simulink model "Progetto_Nostro_Defi"  (Simulink 8.6)
settings: Solver=ode45  StartTime=0.0  StopTime=2.7  RelTol=1e-3
values from neighbouring files (symbols this model uses):
  b = 1e-3    (= 0.001)    [motore_as_param.m]
  Edc = 700    [motore_as_param.m]
  J = Jc+Jm    (= 0.0532)    [motore_as_param.m]
  Kc = Cn/Wn-b    (= 0.178049310978)    [motore_as_param.m]
  Ki_i = 7664    [motore_as_param.m]
  Kp_i = Ki_i*tau_i    (= 32.018926058)    [motore_as_param.m]
  Lr = 123.95e-3    (= 0.12395)    [motore_as_param.m]
  Lrn = Lr    (= 0.12395)    [motore_as_param.m]
  Ls = 123.95e-3    (= 0.12395)    [motore_as_param.m]
  Lsn = Ls    (= 0.12395)    [motore_as_param.m]
  M = 118e-3    (= 0.118)    [motore_as_param.m]
  Mn = M    (= 0.118)    [motore_as_param.m]
  Nn = 1440    [motore_as_param.m]
  p = 2    [motore_as_param.m]
  Rr = 1.137    [motore_as_param.m]
  Rrn = Rr    (= 1.137)    [motore_as_param.m]
  Rs = 2.78    [motore_as_param.m]
  sigma = 1-M*M/(Ls*Lr)    (= 0.0937021444027)    [motore_as_param.m]
  sigman = 1-Mn*Mn/(Lsn*Lrn)    (= 0.0937021444027)    [motore_as_param.m]
  Tc = 200e-6    (= 0.0002)    [motore_as_param.m]
undefined symbols (not defined in the file): Imax, Ki_w, tau_w
libraries: simulink_need_slupdate x2, simulink x1
settings Model: Creator=Gian Filippo Rosi  LastModifiedBy=Gian Filippo Rosi
settings DataIOCC: LimitDataPoints=off  SaveOutput=off  SignalLogging=off  SaveTime=off
settings OptimizationCC: BooleanDataType=off  ExpressionDepthLimit=128  InitFltsAndDblsToZero=on
settings DebuggingCC: SaveWithParameterizedLinksMsg=none  SignalResolutionControl=TryResolveAllWithWarning  SolverPrmCheckMsg=none  MultiTaskDSMMsg=warning  MultiTaskCondExecSysMsg=none  FcnCallInpInsideContextMsg=UseLocalSettings  StateNameClashWarn=none
settings HardwareCC: TargetUnknown=on
settings GRTTargetCC: TargetFcnLib=ansi_tfl_tmw.mat  GeneratePreprocessorConditionals=Use local settings

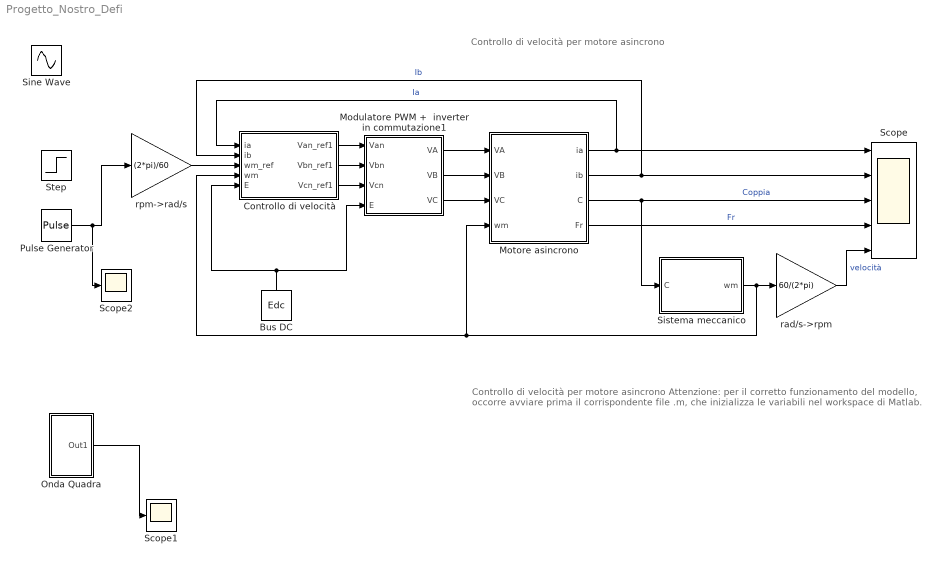
== system Progetto_Nostro_Defi ==
  note: Controllo di velocità per motore asincrono
  note: Controllo di velocità per motore asincrono
      |
      | Attenzione: per il corretto funzionamento del modello, occorre avviare prima
      | il corrispondente file .m, che inizializza le variabili nel workspace di Matlab.
  Bus DC : Constant  Value=Edc
  Controllo di velocità : Subsystem
  Modulatore PWM +  inverter in commutazione1 : Subsystem
  Motore asincrono : Subsystem
  Onda Quadra : Subsystem
  Pulse Generator : DiscretePulseGenerator  PulseType=Time based  Amplitude=2*Nn  PulseWidth=50  PhaseDelay=0.7
  Scope : Scope  NumInputPorts=5
  Scope1 : Scope
  Scope2 : Scope
  Sine Wave : Sin  Amplitude=Nn/4  Frequency=6.28  SampleTime=0
  Sistema meccanico : Subsystem
  Step : Step  Time=0.1+0.6  After=Nn  SampleTime=0
  rad/s->rpm : Gain  Gain=60/(2*pi)  SaturateOnIntegerOverflow=on  OutDataTypeStr=Inherit: Same as input  ParamDataTypeStr=Inherit: Same as input
  rpm->rad/s : Gain  Gain=(2*pi)/60  SaturateOnIntegerOverflow=on  OutDataTypeStr=Inherit: Same as input  ParamDataTypeStr=Inherit: Same as input
  wires:
  Motore asincrono/3(C) -> Scope/3, Sistema meccanico/1(C)  "Coppia"
  Sistema meccanico/1(wm) -> rad/s->rpm/1, Motore asincrono/4(wm), Controllo di velocità/4(wm)
  Motore asincrono/1(ia) -> Controllo di velocità/1(ia), Scope/1  "Ia"
  Motore asincrono/2(ib) -> Scope/2, Controllo di velocità/2(ib)  "Ib"
  Modulatore PWM +  inverter in commutazione1/1(VA) -> Motore asincrono/1(VA)
  Modulatore PWM +  inverter in commutazione1/2(VB) -> Motore asincrono/2(VB)
  Modulatore PWM +  inverter in commutazione1/3(VC) -> Motore asincrono/3(VC)
  Bus DC/1 -> Controllo di velocità/5(E), Modulatore PWM +  inverter in commutazione1/4(E)
  Controllo di velocità/1(Van_ref1) -> Modulatore PWM +  inverter in commutazione1/1(Van)
  Controllo di velocità/2(Vbn_ref1) -> Modulatore PWM +  inverter in commutazione1/2(Vbn)
  rpm->rad/s/1 -> Controllo di velocità/3(wm_ref)
  Controllo di velocità/3(Vcn_ref1) -> Modulatore PWM +  inverter in commutazione1/3(Vcn)
  rad/s->rpm/1 -> Scope/5  "velocità"
  Motore asincrono/4(Fr) -> Scope/4  "Fr"
  Onda Quadra/1(Out1) -> Scope1/1
  Pulse Generator/1 -> Scope2/1, rpm->rad/s/1

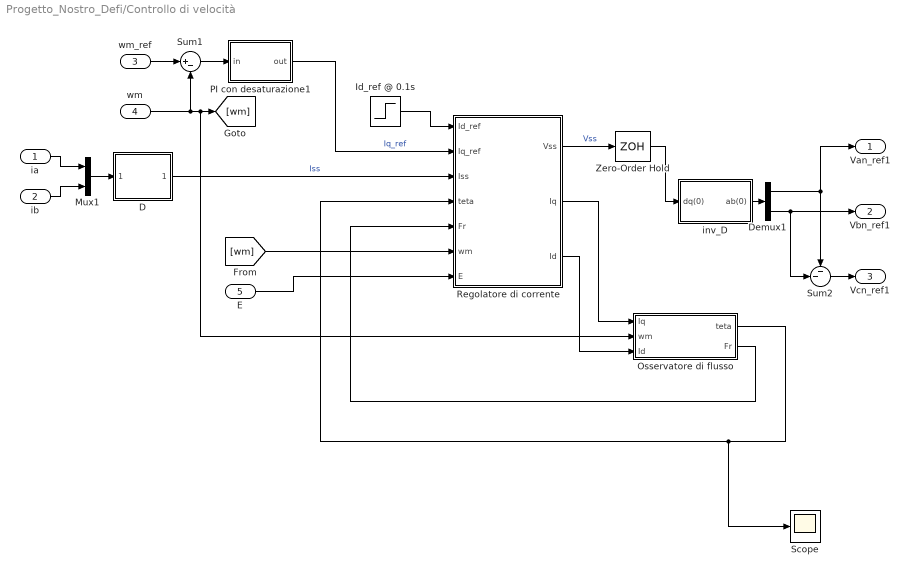
== system Progetto_Nostro_Defi/Controllo di velocità ==
  ia : Inport
  ib : Inport  Port=2
  wm_ref : Inport  Port=3
  wm : Inport  Port=4
  E : Inport  Port=5
  D : Subsystem
  Demux1 : Demux  Outputs=2
  Id_ref @ 0.1s : Step  Time=0.1  After=7.644  SampleTime=0
  Mux1 : Mux  Inputs=2
  Osservatore di flusso : Subsystem
  PI con desaturazione1 : Subsystem  mask{UB=Imax, LB=-Imax, tau=tau_w, Kp=Ki_w*tau_w}
      mask prompts: UB "Limite superiore"; LB "Limte inferiore"; tau "Tau (s)"
      mask Display: fprintf('PI\nantiwindup')
  Regolatore di corrente : Subsystem
  Scope : Scope
  Sum1 : Sum  Inputs=|+-
  Sum2 : Sum  Inputs=--|
  Zero-Order Hold : ZeroOrderHold  SampleTime=Tc
  inv_D : Subsystem
  Van_ref1 : Outport
  Vbn_ref1 : Outport  Port=2
  Vcn_ref1 : Outport  Port=3
  wires:
  inv_D/1(ab(0)) -> Demux1/1
  Sum2/1 -> Vcn_ref1/1
  Demux1/1 -> Sum2/1, Van_ref1/1
  Demux1/2 -> Sum2/2, Vbn_ref1/1
  Mux1/1 -> D/1(ab(c))
  ia/1 -> Mux1/1
  ib/1 -> Mux1/2
  D/1(dq(0)) -> Regolatore di corrente/3(Iss)  "Iss"
  Regolatore di corrente/1(Vss) -> Zero-Order Hold/1  "Vss"
  Osservatore di flusso/2(Fr) -> Regolatore di corrente/5(Fr)
  Osservatore di flusso/1(teta) -> Scope/1, Regolatore di corrente/4(teta)
  [wm] -> Regolatore di corrente/6(wm)
  E/1 -> Regolatore di corrente/7(E)
  wm/1 -> Osservatore di flusso/2(wm), [wm], Sum1/2
  wm_ref/1 -> Sum1/1
  Sum1/1 -> PI con desaturazione1/1(in)
  PI con desaturazione1/1(out) -> Regolatore di corrente/2(Iq_ref)  "Iq_ref"
  Zero-Order Hold/1 -> inv_D/1(dq(0))
  Id_ref @ 0.1s/1 -> Regolatore di corrente/1(Id_ref)
  Regolatore di corrente/2(Iq) -> Osservatore di flusso/1(Iq)
  Regolatore di corrente/3(Id) -> Osservatore di flusso/3(Id)

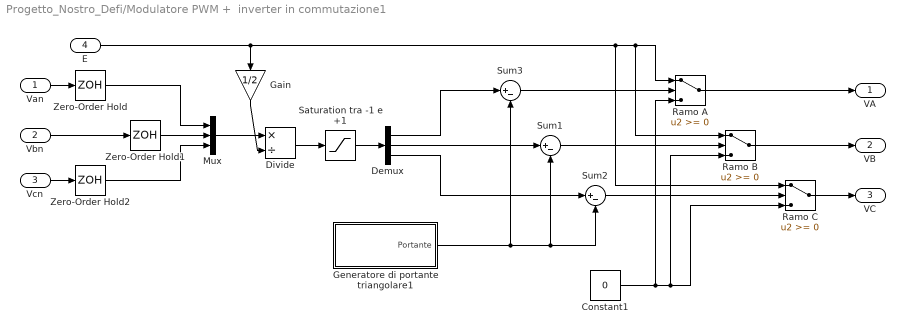
== system Progetto_Nostro_Defi/Modulatore PWM +  inverter in commutazione1 ==
  Van : Inport
  Vbn : Inport  Port=2
  Vcn : Inport  Port=3
  E : Inport  Port=4
  Constant1 : Constant  Value=0
  Demux : Demux  Outputs=3
  Divide : Product  Inputs=*/
  Gain : Gain  Gain=1/2
  Generatore di portante triangolare1 : Subsystem
  Mux : Mux  Inputs=3
  Ramo A : Switch
  Ramo B : Switch
  Ramo C : Switch
  Saturation tra -1 e +1 : Saturate  UpperLimit=1  LowerLimit=-1
  Sum1 : Sum  Inputs=|+-
  Sum2 : Sum  Inputs=|+-
  Sum3 : Sum  Inputs=|+-
  Zero-Order Hold : ZeroOrderHold  SampleTime=Tc
  Zero-Order Hold1 : ZeroOrderHold  SampleTime=Tc
  Zero-Order Hold2 : ZeroOrderHold  SampleTime=Tc
  VA : Outport
  VB : Outport  Port=2
  VC : Outport  Port=3
  wires:
  Van/1 -> Zero-Order Hold/1
  Vbn/1 -> Zero-Order Hold1/1
  Vcn/1 -> Zero-Order Hold2/1
  Mux/1 -> Divide/1
  E/1 -> Ramo A/1, Ramo B/1, Ramo C/1, Gain/1
  Divide/1 -> Saturation tra -1 e +1/1
  Saturation tra -1 e +1/1 -> Demux/1
  Sum3/1 -> Ramo A/2
  Constant1/1 -> Ramo A/3, Ramo C/3, Ramo B/3
  Ramo A/1 -> VA/1
  Ramo C/1 -> VC/1
  Ramo B/1 -> VB/1
  Sum1/1 -> Ramo B/2
  Sum2/1 -> Ramo C/2
  Generatore di portante triangolare1/1(Portante) -> Sum1/2, Sum2/2, Sum3/2
  Demux/1 -> Sum3/1
  Demux/2 -> Sum1/1
  Demux/3 -> Sum2/1
  Gain/1 -> Divide/2
  Zero-Order Hold/1 -> Mux/1
  Zero-Order Hold1/1 -> Mux/2
  Zero-Order Hold2/1 -> Mux/3

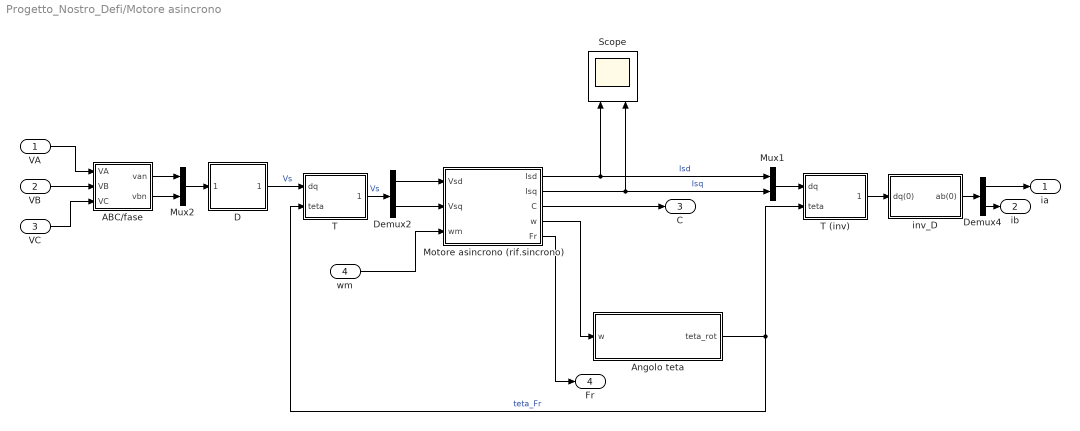
== system Progetto_Nostro_Defi/Motore asincrono ==
  VA : Inport
  VB : Inport  Port=2
  VC : Inport  Port=3
  wm : Inport  Port=4
  ABC/fase : Subsystem
  Angolo teta : Subsystem
      mask Display:
      | dpoly([1],[1 0],'s');
      | port_label('output',1,'teta_rot');
      | port_label('input',1,'w');
  D : Subsystem
  Demux2 : Demux  Outputs=2
  Demux4 : Demux  Outputs=2
  Motore asincrono (rif.sincrono) : Subsystem
  Mux1 : Mux  Inputs=2
  Mux2 : Mux  Inputs=2
  Scope : Scope  NumInputPorts=2
  T : Subsystem
  T (inv) : Subsystem
  inv_D : Subsystem
  ia : Outport
  ib : Outport  Port=2
  C : Outport  Port=3
  Fr : Outport  Port=4
  wires:
  VA/1 -> ABC/fase/1(VA)
  VB/1 -> ABC/fase/2(VB)
  VC/1 -> ABC/fase/3(VC)
  ABC/fase/1(van) -> Mux2/1
  ABC/fase/2(vbn) -> Mux2/2
  Mux2/1 -> D/1(ab(c))
  inv_D/1(ab(0)) -> Demux4/1
  Demux4/1 -> ia/1
  Demux4/2 -> ib/1
  D/1(dq(0)) -> T/1(dq)  "Vs"
  T/1(dq(teta)) -> Demux2/1  "Vs"
  Mux1/1 -> T (inv)/1(dq)
  Demux2/1 -> Motore asincrono (rif.sincrono)/1(Vsd)
  Demux2/2 -> Motore asincrono (rif.sincrono)/2(Vsq)
  wm/1 -> Motore asincrono (rif.sincrono)/3(wm)
  Motore asincrono (rif.sincrono)/4(w) -> Angolo teta/1(w)
  Motore asincrono (rif.sincrono)/1(Isd) -> Scope/1, Mux1/1  "Isd"
  Motore asincrono (rif.sincrono)/2(Isq) -> Scope/2, Mux1/2  "Isq"
  Motore asincrono (rif.sincrono)/3(C) -> C/1
  T (inv)/1(dq(teta)) -> inv_D/1(dq(0))
  Angolo teta/1(teta_rot) -> T/2(teta), T (inv)/2(teta)  "teta_Fr"
  Motore asincrono (rif.sincrono)/5(Fr) -> Fr/1

== system Progetto_Nostro_Defi/Onda Quadra ==
  Add : Sum
  Pulse Generator : DiscretePulseGenerator  PulseType=Time based  Amplitude=-Nn  PulseWidth=50  PhaseDelay=1.7
  Pulse Generator1 : DiscretePulseGenerator  PulseType=Time based  Amplitude=Nn  PulseWidth=50  PhaseDelay=0.7
  Out1 : Outport
  wires:
  Pulse Generator1/1 -> Add/1
  Pulse Generator/1 -> Add/2
  Add/1 -> Out1/1

== system Progetto_Nostro_Defi/Sistema meccanico ==
  C : Inport
  Gain : Gain  Gain=Kc
  Sum : Sum  Inputs=|+-  SaturateOnIntegerOverflow=on  InputSameDT=on  OutDataTypeStr=Inherit: Same as first input
  Transfer Fcn : TransferFcn  Denominator=[J b]
  wm : Outport
  wires:
  C/1 -> Sum/1
  Sum/1 -> Transfer Fcn/1
  Transfer Fcn/1 -> wm/1, Gain/1  "wm"
  Gain/1 -> Sum/2  "Cr"

== system Progetto_Nostro_Defi/Controllo di velocità/D ==
  ab(c) : Inport
  Gain : Gain  Gain=[1 0; 1/sqrt(3) 2/sqrt(3)]  Multiplication=Matrix(K*u)
  dq(0) : Outport
  wires:
  ab(c)/1 -> Gain/1
  Gain/1 -> dq(0)/1

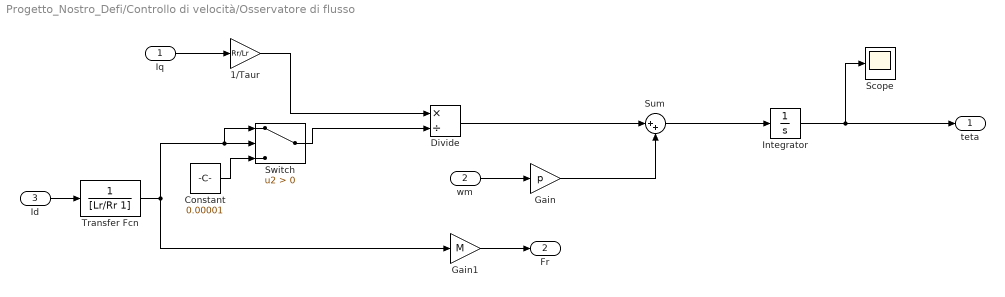
== system Progetto_Nostro_Defi/Controllo di velocità/Osservatore di flusso ==
  Iq : Inport
  wm : Inport  Port=2
  Id : Inport  Port=3
  1/Taur : Gain  Gain=Rr/Lr
  Constant : Constant  Value=0.00001
  Divide : Product  Inputs=*/
  Gain : Gain  Gain=p
  Gain1 : Gain  Gain=M
  Integrator : Integrator  WrapState=on  WrappedStateUpperValue=2*pi  WrappedStateLowerValue=-2*pi
  Scope : Scope
  Sum : Sum  Inputs=|++
  Switch : Switch  Criteria=u2 > Threshold
  Transfer Fcn : TransferFcn  Denominator=[Lr/Rr 1]
  teta : Outport
  Fr : Outport  Port=2
  wires:
  Iq/1 -> 1/Taur/1
  1/Taur/1 -> Divide/1
  wm/1 -> Gain/1
  Gain/1 -> Sum/2
  Gain1/1 -> Fr/1
  Id/1 -> Transfer Fcn/1
  Switch/1 -> Divide/2
  Transfer Fcn/1 -> Gain1/1, Switch/1, Switch/2
  Constant/1 -> Switch/3
  Sum/1 -> Integrator/1
  Integrator/1 -> Scope/1, teta/1
  Divide/1 -> Sum/1

== system Progetto_Nostro_Defi/Controllo di velocità/PI con desaturazione1 ==
  in : Inport
  Gain : Gain  Gain=Kp
  Saturation : Saturate  UpperLimit=UB  LowerLimit=LB
  Sum2 : Sum  Inputs=|++
  Transfer Fcn : TransferFcn  Denominator=[tau 1]
  out : Outport
  wires:
  Gain/1 -> Sum2/1
  Transfer Fcn/1 -> Sum2/2
  Sum2/1 -> Saturation/1
  Saturation/1 -> Transfer Fcn/1, out/1
  in/1 -> Gain/1

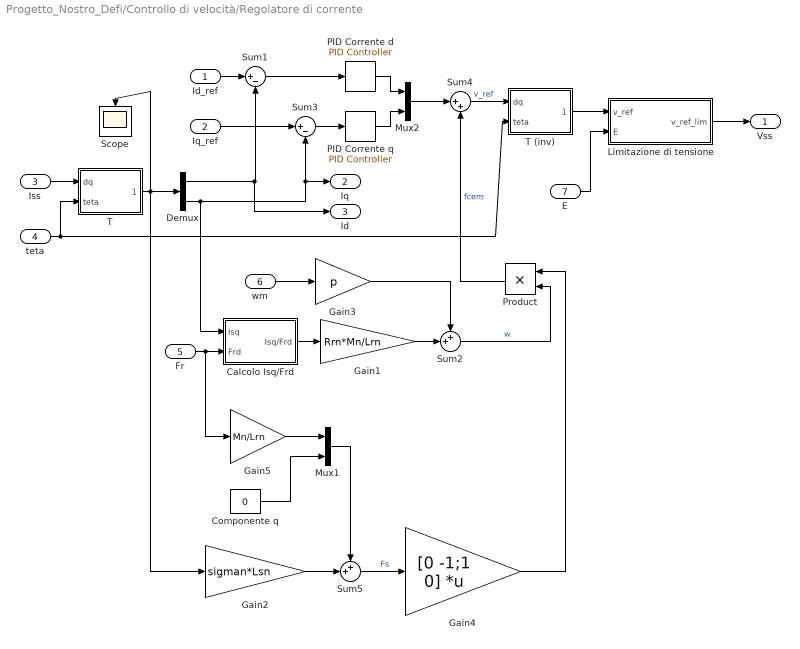
== system Progetto_Nostro_Defi/Controllo di velocità/Regolatore di corrente ==
  Id_ref : Inport
  Iq_ref : Inport  Port=2
  Iss : Inport  Port=3
  teta : Inport  Port=4
  Fr : Inport  Port=5
  wm : Inport  Port=6
  E : Inport  Port=7
  Calcolo Isq/Frd : Subsystem
  Componente q : Constant  Value=0
  Demux : Demux  Outputs=2
  Gain1 : Gain  Gain=Rrn*Mn/Lrn  SaturateOnIntegerOverflow=on  OutDataTypeStr=Inherit: Same as input  ParamDataTypeStr=Inherit: Same as input
  Gain2 : Gain  Gain=sigman*Lsn
  Gain3 : Gain  Gain=p  SaturateOnIntegerOverflow=on  OutDataTypeStr=Inherit: Same as input  ParamDataTypeStr=Inherit: Same as input
  Gain4 : Gain  Gain=[0 -1;1 0]  Multiplication=Matrix(K*u)  SaturateOnIntegerOverflow=on  OutDataTypeStr=Inherit: Same as input  ParamDataTypeStr=Inherit: Same as input
  Gain5 : Gain  Gain=Mn/Lrn
  Limitazione di tensione : Subsystem
  Mux1 : Mux  Inputs=2
  Mux2 : Mux  Inputs=2
  PID Corrente d : simulink_need_slupdate/PID Controller  P=Kp_i  I=Ki_i  D=0
  PID Corrente q : simulink_need_slupdate/PID Controller  P=Kp_i  I=Ki_i  D=0
  Product : Product  RndMeth=Zero
  Scope : Scope
  Sum1 : Sum  Inputs=|+-
  Sum2 : Sum  Inputs=++|
  Sum3 : Sum  Inputs=|+-
  Sum4 : Sum  Inputs=|++
  Sum5 : Sum  Inputs=++|  SaturateOnIntegerOverflow=on  InputSameDT=on  OutDataTypeStr=Inherit: Same as first input
  T : Subsystem
  T (inv) : Subsystem
  Vss : Outport
  Iq : Outport  Port=2
  Id : Outport  Port=3
  wires:
  Iss/1 -> T/1(dq)
  T/1(dq(teta)) -> Demux/1, Scope/1, Gain2/1
  Demux/1 -> Id/1, Sum1/2
  Demux/2 -> Iq/1, Sum3/2, Calcolo Isq/Frd/1(Isq)
  Sum1/1 -> PID Corrente d/1
  Sum3/1 -> PID Corrente q/1
  PID Corrente d/1 -> Mux2/1
  PID Corrente q/1 -> Mux2/2
  Mux2/1 -> Sum4/1
  Sum4/1 -> T (inv)/1(dq)  "v_ref"
  Product/1 -> Sum4/2  "fcem"
  Id_ref/1 -> Sum1/1
  Iq_ref/1 -> Sum3/1
  teta/1 -> T/2(teta), T (inv)/2(teta)
  Sum2/1 -> Product/2  "w"
  wm/1 -> Gain3/1
  Calcolo Isq/Frd/1(Isq/Frd) -> Gain1/1
  Fr/1 -> Calcolo Isq/Frd/2(Frd), Gain5/1
  Gain4/1 -> Product/1
  Sum5/1 -> Gain4/1  "Fs"
  Componente q/1 -> Mux1/2
  Gain5/1 -> Mux1/1
  Gain1/1 -> Sum2/2
  Gain3/1 -> Sum2/1
  Gain2/1 -> Sum5/2
  Mux1/1 -> Sum5/1
  T (inv)/1(dq(teta)) -> Limitazione di tensione/1(v_ref)
  Limitazione di tensione/1(v_ref_lim) -> Vss/1
  E/1 -> Limitazione di tensione/2(E)

== system Progetto_Nostro_Defi/Controllo di velocità/inv_D ==
  dq(0) : Inport
  Gain : Gain  Gain=[1 0; -1/2 sqrt(3)/2]  Multiplication=Matrix(K*u)
  ab(0) : Outport
  wires:
  dq(0)/1 -> Gain/1
  Gain/1 -> ab(0)/1

== system Progetto_Nostro_Defi/Modulatore PWM +  inverter in commutazione1/Generatore di portante triangolare1 ==
  note: Nell'integratore settare la
      | condizione iniziale a +1
  note: Questo blocco genera un'onda triangolare da +1 e -1, di periodo Tc.
  Constant : Constant  Value=4/Tc
  Integrator Initial condition: +1 : Integrator  InitialCondition=1
  Pulse Generator : DiscretePulseGenerator  PulseType=Time based  Amplitude=8/Tc  Period=Tc  PulseWidth=50
  Sum : Sum  Inputs=-+
  Portante : Outport
  wires:
  Sum/1 -> Integrator Initial condition: +1/1
  Pulse Generator/1 -> Sum/1
  Constant/1 -> Sum/2
  Integrator Initial condition: +1/1 -> Portante/1

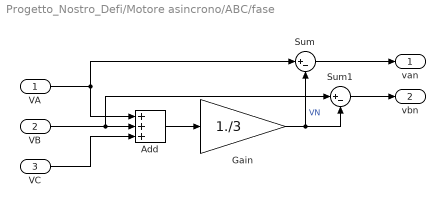
== system Progetto_Nostro_Defi/Motore asincrono/ABC/fase ==
  VA : Inport
  VB : Inport  Port=2
  VC : Inport  Port=3
  Add : Sum  Inputs=+++
  Gain : Gain  Gain=1./3
  Sum : Sum  Inputs=|+-
  Sum1 : Sum  Inputs=|+-
  van : Outport
  vbn : Outport  Port=2
  wires:
  VA/1 -> Add/1, Sum/1
  VB/1 -> Add/2, Sum1/1
  VC/1 -> Add/3
  Add/1 -> Gain/1
  Gain/1 -> Sum/2, Sum1/2  "VN"
  Sum/1 -> van/1
  Sum1/1 -> vbn/1

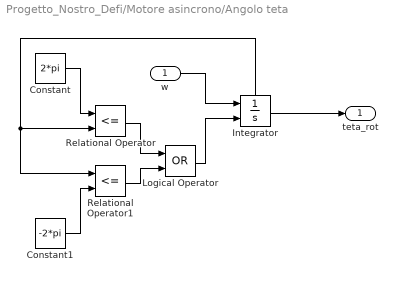
== system Progetto_Nostro_Defi/Motore asincrono/Angolo teta ==
  w : Inport
  Constant : Constant  Value=2*pi
  Constant1 : Constant  Value=-2*pi
  Integrator : Integrator  ExternalReset=rising  ShowStatePort=on
  Logical Operator : Logic  Operator=OR  AllPortsSameDT=off  OutDataTypeStr=boolean
  Relational Operator : RelationalOperator  Operator=<=  OutDataTypeStr=boolean
  Relational Operator1 : RelationalOperator  Operator=<=  OutDataTypeStr=boolean
  teta_rot : Outport
  wires:
  Integrator/1 -> teta_rot/1
  Logical Operator/1 -> Integrator/2
  Relational Operator/1 -> Logical Operator/1
  Relational Operator1/1 -> Logical Operator/2
  w/1 -> Integrator/1
  Integrator/State -> Relational Operator1/1, Relational Operator/2
  Constant/1 -> Relational Operator/1
  Constant1/1 -> Relational Operator1/2

== system Progetto_Nostro_Defi/Motore asincrono/D ==
  ab(c) : Inport
  Gain : Gain  Gain=[1 0; 1/sqrt(3) 2/sqrt(3)]  Multiplication=Matrix(K*u)
  dq(0) : Outport
  wires:
  ab(c)/1 -> Gain/1
  Gain/1 -> dq(0)/1

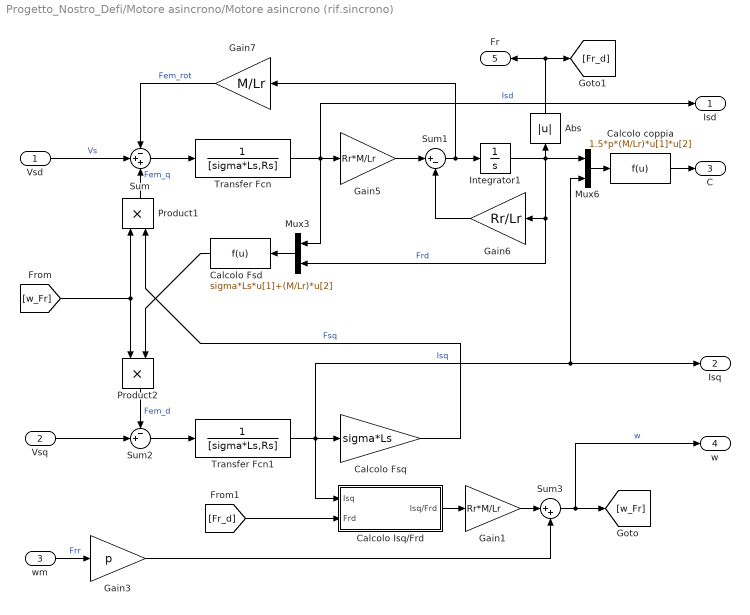
== system Progetto_Nostro_Defi/Motore asincrono/Motore asincrono (rif.sincrono) ==
  Vsd : Inport
  Vsq : Inport  Port=2
  wm : Inport  Port=3
  Abs : Abs
  Calcolo Fsd : Fcn  Expr=sigma*Ls*u[1]+(M/Lr)*u[2]
  Calcolo Fsq : Gain  Gain=sigma*Ls  SaturateOnIntegerOverflow=on  OutDataTypeStr=Inherit: Same as input  ParamDataTypeStr=Inherit: Same as input
  Calcolo Isq/Frd : Subsystem
  Calcolo coppia : Fcn  Expr=1.5*p*(M/Lr)*u[1]*u[2]
  Gain1 : Gain  Gain=Rr*M/Lr  SaturateOnIntegerOverflow=on  OutDataTypeStr=Inherit: Same as input  ParamDataTypeStr=Inherit: Same as input
  Gain3 : Gain  Gain=p  SaturateOnIntegerOverflow=on  OutDataTypeStr=Inherit: Same as input  ParamDataTypeStr=Inherit: Same as input
  Gain5 : Gain  Gain=Rr*M/Lr
  Gain6 : Gain  Gain=Rr/Lr
  Gain7 : Gain  Gain=M/Lr
  Integrator1 : Integrator
  Mux3 : Mux  Inputs=2
  Mux6 : Mux  Inputs=2
  Product1 : Product  RndMeth=Zero
  Product2 : Product  RndMeth=Zero
  Sum : Sum  Inputs=-++
  Sum1 : Sum  Inputs=|+-
  Sum2 : Sum  Inputs=-+|
  Sum3 : Sum  Inputs=|++
  Transfer Fcn : TransferFcn  Denominator=[sigma*Ls,Rs]
  Transfer Fcn1 : TransferFcn  Denominator=[sigma*Ls,Rs]
  Isd : Outport
  Isq : Outport  Port=2
  C : Outport  Port=3
  w : Outport  Port=4
  Fr : Outport  Port=5
  wires:
  Mux6/1 -> Calcolo coppia/1
  Vsd/1 -> Sum/2  "Vs"
  Sum/1 -> Transfer Fcn/1
  Transfer Fcn/1 -> Gain5/1, Mux3/1, Isd/1  "Isd"
  Gain5/1 -> Sum1/1
  Sum1/1 -> Integrator1/1, Gain7/1
  Integrator1/1 -> Mux6/1, Mux3/2, Gain6/1, Abs/1  "Frd"
  Gain6/1 -> Sum1/2
  Sum2/1 -> Transfer Fcn1/1
  Mux3/1 -> Calcolo Fsd/1
  Transfer Fcn1/1 -> Calcolo Fsq/1, Calcolo Isq/Frd/1(Isq), Mux6/2, Isq/1  "Isq"
  Sum3/1 -> [w_Fr], w/1  "w"
  Gain7/1 -> Sum/1  "Fem_rot"
  Product1/1 -> Sum/3  "Fem_q"
  Product2/1 -> Sum2/1  "Fem_d"
  Calcolo Fsq/1 -> Product1/2  "Fsq"
  [w_Fr] -> Product1/1, Product2/1
  wm/1 -> Gain3/1  "Frr"
  Calcolo Isq/Frd/1(Isq/Frd) -> Gain1/1
  Gain1/1 -> Sum3/1
  Gain3/1 -> Sum3/2
  [Fr_d] -> Calcolo Isq/Frd/2(Frd)
  Vsq/1 -> Sum2/2
  Calcolo coppia/1 -> C/1
  Abs/1 -> [Fr_d], Fr/1
  Calcolo Fsd/1 -> Product2/2

== system Progetto_Nostro_Defi/Motore asincrono/T ==
  dq : Inport
  teta : Inport  Port=2
  Demux : Demux  Outputs=2
  Fcn : Fcn  Expr=cos(u[3])*u[1]+sin(u[3])*u[2]
  Fcn1 : Fcn  Expr=-sin(u[3])*u[1]+cos(u[3])*u[2]
  Mux : Mux  Inputs=3
  Mux1 : Mux  Inputs=2
  dq(teta) : Outport
  wires:
  dq/1 -> Demux/1
  Demux/1 -> Mux/1
  Demux/2 -> Mux/2
  teta/1 -> Mux/3
  Mux/1 -> Fcn/1, Fcn1/1
  Fcn/1 -> Mux1/1
  Fcn1/1 -> Mux1/2
  Mux1/1 -> dq(teta)/1

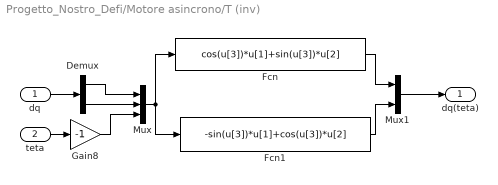
== system Progetto_Nostro_Defi/Motore asincrono/T (inv) ==
  dq : Inport
  teta : Inport  Port=2
  Demux : Demux  Outputs=2
  Fcn : Fcn  Expr=cos(u[3])*u[1]+sin(u[3])*u[2]
  Fcn1 : Fcn  Expr=-sin(u[3])*u[1]+cos(u[3])*u[2]
  Gain8 : Gain  Gain=-1
  Mux : Mux  Inputs=3
  Mux1 : Mux  Inputs=2
  dq(teta) : Outport
  wires:
  dq/1 -> Demux/1
  Demux/1 -> Mux/1
  Demux/2 -> Mux/2
  teta/1 -> Gain8/1
  Mux/1 -> Fcn/1, Fcn1/1
  Fcn/1 -> Mux1/1
  Fcn1/1 -> Mux1/2
  Mux1/1 -> dq(teta)/1
  Gain8/1 -> Mux/3

== system Progetto_Nostro_Defi/Motore asincrono/inv_D ==
  dq(0) : Inport
  Gain : Gain  Gain=[1 0; -1/2 sqrt(3)/2]  Multiplication=Matrix(K*u)
  ab(0) : Outport
  wires:
  dq(0)/1 -> Gain/1
  Gain/1 -> ab(0)/1

== system Progetto_Nostro_Defi/Controllo di velocità/Regolatore di corrente/Calcolo Isq/Frd ==
  Isq : Inport
  Frd : Inport  Port=2
  Constant : Constant  Value=0
  Constant1 : Constant
  Product : Product  Inputs=*/  RndMeth=Zero
  Switch : Switch  Criteria=u2 > Threshold  Threshold=0.001
  Switch1 : Switch  Criteria=u2 > Threshold  Threshold=.001
  Isq/Frd : Outport
  wires:
  Constant/1 -> Switch/3
  Product/1 -> Switch/1
  Constant1/1 -> Switch1/3
  Switch/1 -> Isq/Frd/1
  Frd/1 -> Switch1/1, Switch1/2, Switch/2
  Isq/1 -> Product/1
  Switch1/1 -> Product/2

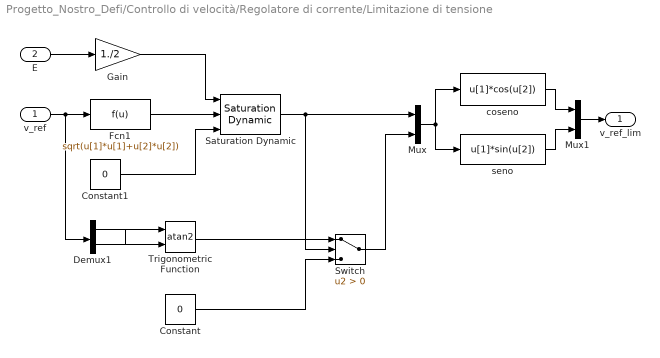
== system Progetto_Nostro_Defi/Controllo di velocità/Regolatore di corrente/Limitazione di tensione ==
  v_ref : Inport
  E : Inport  Port=2
  Constant : Constant  Value=0
  Constant1 : Constant  Value=0
  Demux1 : Demux  Outputs=2
  Fcn1 : Fcn  Expr=sqrt(u[1]*u[1]+u[2]*u[2])
  Gain : Gain  Gain=1./2
  Mux : Mux  Inputs=2
  Mux1 : Mux  Inputs=2
  Saturation Dynamic : simulink/Discontinuities/Saturation Dynamic  OutMin=[]  OutMax=[]  OutDataTypeStr=Inherit: Same as second input  OutDataType=fixdt(1, 16)  OutScaling=2^-10  DoSatur=off
  Switch : Switch  Criteria=u2 > Threshold
  Trigonometric Function : Trigonometry  Operator=atan2
  coseno : Fcn  Expr=u[1]*cos(u[2])
  seno : Fcn  Expr=u[1]*sin(u[2])
  v_ref_lim : Outport
  wires:
  v_ref/1 -> Fcn1/1, Demux1/1
  Constant/1 -> Switch/3
  Demux1/2 -> Trigonometric Function/1
  Demux1/1 -> Trigonometric Function/2
  Trigonometric Function/1 -> Switch/1
  Switch/1 -> Mux/2
  Fcn1/1 -> Saturation Dynamic/2
  E/1 -> Gain/1
  Gain/1 -> Saturation Dynamic/1
  Constant1/1 -> Saturation Dynamic/3
  Saturation Dynamic/1 -> Switch/2, Mux/1
  Mux/1 -> coseno/1, seno/1
  coseno/1 -> Mux1/1
  seno/1 -> Mux1/2
  Mux1/1 -> v_ref_lim/1

== system Progetto_Nostro_Defi/Controllo di velocità/Regolatore di corrente/T ==
  dq : Inport
  teta : Inport  Port=2
  Demux : Demux  Outputs=2
  Fcn : Fcn  Expr=cos(u[3])*u[1]+sin(u[3])*u[2]
  Fcn1 : Fcn  Expr=-sin(u[3])*u[1]+cos(u[3])*u[2]
  Mux : Mux  Inputs=3
  Mux1 : Mux  Inputs=2
  dq(teta) : Outport
  wires:
  dq/1 -> Demux/1
  Demux/1 -> Mux/1
  Demux/2 -> Mux/2
  teta/1 -> Mux/3
  Mux/1 -> Fcn/1, Fcn1/1
  Fcn/1 -> Mux1/1
  Fcn1/1 -> Mux1/2
  Mux1/1 -> dq(teta)/1

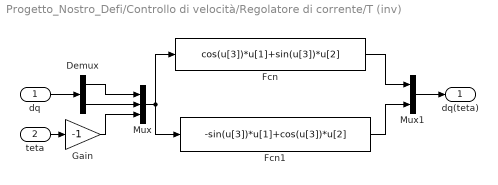
== system Progetto_Nostro_Defi/Controllo di velocità/Regolatore di corrente/T (inv) ==
  dq : Inport
  teta : Inport  Port=2
  Demux : Demux  Outputs=2
  Fcn : Fcn  Expr=cos(u[3])*u[1]+sin(u[3])*u[2]
  Fcn1 : Fcn  Expr=-sin(u[3])*u[1]+cos(u[3])*u[2]
  Gain : Gain  Gain=-1
  Mux : Mux  Inputs=3
  Mux1 : Mux  Inputs=2
  dq(teta) : Outport
  wires:
  dq/1 -> Demux/1
  Demux/1 -> Mux/1
  Demux/2 -> Mux/2
  teta/1 -> Gain/1
  Mux/1 -> Fcn/1, Fcn1/1
  Fcn/1 -> Mux1/1
  Fcn1/1 -> Mux1/2
  Mux1/1 -> dq(teta)/1
  Gain/1 -> Mux/3

== system Progetto_Nostro_Defi/Motore asincrono/Motore asincrono (rif.sincrono)/Calcolo Isq/Frd ==
  Isq : Inport
  Frd : Inport  Port=2
  Constant : Constant  Value=0
  Constant1 : Constant
  Product : Product  Inputs=*/  RndMeth=Zero
  Switch : Switch  Criteria=u2 > Threshold  Threshold=0.001
  Switch1 : Switch  Criteria=u2 > Threshold  Threshold=.001
  Isq/Frd : Outport
  wires:
  Constant/1 -> Switch/3
  Product/1 -> Switch/1
  Constant1/1 -> Switch1/3
  Switch/1 -> Isq/Frd/1
  Frd/1 -> Switch1/1, Switch1/2, Switch/2
  Isq/1 -> Product/1
  Switch1/1 -> Product/2
